simulink model "My_1st_Model_Fallschrimspringer"  (R2024b)
settings: Solver=VariableStepAuto  StartTime=0.0  StopTime=400  RelTol=1e-3
model workspace: external: MATLAB File /home/arash/Matlab/2-Einführungsbeispiel-zur-Modellierung/Implementierungsvarianten_FMS/Fallschirmspringer/My_Try/Y_Parameter_Fallschirmspringer.m (data not in the file)
values from neighbouring files (symbols this model uses):
  A_FS = 30    [Y_Parameter_Fallschirmspringer.m]
  A_S = 0.5    [Y_Parameter_Fallschirmspringer.m]
  cW = 1.3    [Y_Parameter_Fallschirmspringer.m]
  g = 9.81    [Y_Parameter_Fallschirmspringer.m]
  h_0 = 3000    [Y_Parameter_Fallschirmspringer.m]
  h_1 = 1500    [Y_Parameter_Fallschirmspringer.m]
  m = 85    [Y_Parameter_Fallschirmspringer.m]
  rho = 1.2    [Y_Parameter_Fallschirmspringer.m]
settings Model: Creator=arash  LastModifiedBy=arash

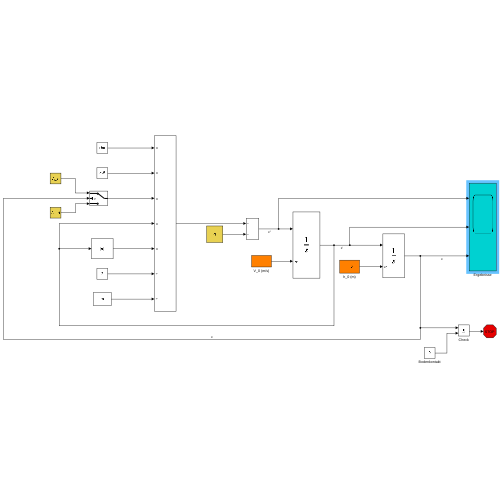
[thumbnail: Simulink's stored preview of the top-level diagram]
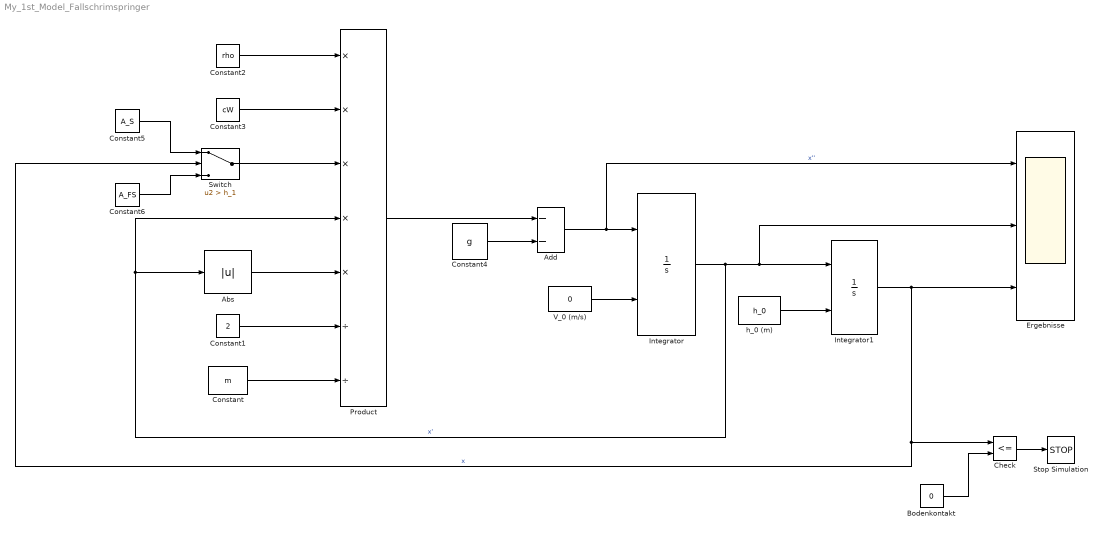
== system My_1st_Model_Fallschrimspringer ==
  Abs : Abs  SaturateOnIntegerOverflow=off
  Add : Sum  Inputs=--
  Bodenkontakt : Constant  Value=0
  Check : RelationalOperator  Operator=<=  OutDataTypeStr=boolean  RndMeth=Simplest  InputSameDT=off
  Constant : Constant  Value=m
  Constant1 : Constant  Value=2
  Constant2 : Constant  Value=rho
  Constant3 : Constant  Value=cW
  Constant4 : Constant  Value=g
  Constant5 : Constant  Value=A_S
  Constant6 : Constant  Value=A_FS
  Ergebnisse : Scope  NumInputPorts=3
  Integrator : Integrator  InitialConditionSource=external
  Integrator1 : Integrator  InitialConditionSource=external
  Product : Product  Inputs=*****//
  Stop Simulation : Stop
  Switch : Switch  Criteria=u2 > Threshold  Threshold=h_1  SaturateOnIntegerOverflow=off  InputSameDT=off
  V_0 (m/s) : Constant  Value=0
  h_0 (m) : Constant  Value=h_0
  wires:
  Constant/1 -> Product/7
  Constant1/1 -> Product/6
  Constant2/1 -> Product/1
  Constant3/1 -> Product/2
  Switch/1 -> Product/3
  Product/1 -> Add/1
  Constant4/1 -> Add/2
  Add/1 -> Ergebnisse/1, Integrator/1  "x''"
  V_0 (m/s)/1 -> Integrator/2
  Integrator/1 -> Product/4, Abs/1, Ergebnisse/2, Integrator1/1  "x'"
  h_0 (m)/1 -> Integrator1/2
  Integrator1/1 -> Switch/2, Check/1, Ergebnisse/3  "x"
  Abs/1 -> Product/5
  Constant5/1 -> Switch/1
  Constant6/1 -> Switch/3
  Bodenkontakt/1 -> Check/2
  Check/1 -> Stop Simulation/1
